simulink model "chap6_5sim"  (Simulink 6.3)
settings: Solver=ode45  StartTime=0.0  StopTime=15  RelTol=1e-3
settings Model: LastModifiedBy=Administrator  ExtModeTrigMode=oneshot  ExtModeArmWhenConnect=off  StrictBusMsg=None
settings DataIOCC: LimitDataPoints=off  SignalLoggingName=sigsOut
settings OptimizationCC: BooleanDataType=off
settings DebuggingCC: SolverPrmCheckMsg=none
settings HardwareCC: TargetUnknown=on

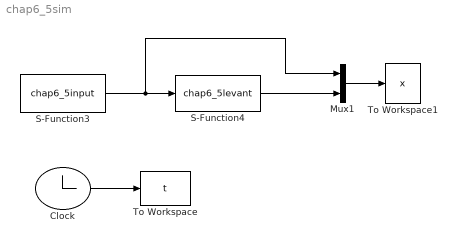
== system chap6_5sim ==
  Clock : Clock
  Mux1 : Mux  Inputs=2
  S-Function3 : S-Function  FunctionName=chap6_5input
  S-Function4 : S-Function  FunctionName=chap6_5levant
  To Workspace : ToWorkspace  VariableName=t  SampleTime=-1  SaveFormat=Array
  To Workspace1 : ToWorkspace  VariableName=x  SampleTime=-1  SaveFormat=Array
  wires:
  Clock/1 -> To Workspace/1
  S-Function3/1 -> S-Function4/1, Mux1/1
  S-Function4/1 -> Mux1/2
  Mux1/1 -> To Workspace1/1
